simulink model "Van_der_Pol"  (Simulink 9.1)
settings: Solver=VariableStepAuto  StartTime=0.0  StopTime=20  RelTol=1e-3
settings Model: SuppressorTable=22 serialization::archive 11 0 6 0 0 0 0 0  Creator=BEAR  LastModifiedBy=BEAR
settings DataIOCC: SaveFormat=Dataset
settings OptimizationCC: LifeSpan=auto
settings DebuggingCC: UnderspecifiedInitializationDetection=Simplified  MergeDetectMultiDrivingBlocksExec=error  SFUnexpectedBacktrackingDiag=error  SFNoUnconditionalDefaultTransitionDiag=error  SFExecutionAtInitializationDiag=warning
settings HardwareCC: ProdBitPerPointer=64  ProdBitPerSizeT=64  ProdBitPerPtrDiffT=64  ProdLargestAtomicFloat=Float  ProdIntDivRoundTo=Zero  ProdEndianess=LittleEndian  ProdWordSize=64  ProdHWDeviceType=Intel->x86-64 (Windows64)
settings ModelReferenceCC: PropagateSignalLabelsOutOfModel=on
settings CodeAppCC: StateflowObjectComments=off
settings GRTTargetCC: TargetLangStandard=C99 (ISO)  CombineOutputUpdateFcns=on  GRTInterface=off
settings ConfigComp: CovMetricSettings=dwe  CovHtmlReporting=off  CovSaveCumulativeToWorkspaceVar=off  CovSaveSingleToWorkspaceVar=off  CovExternalEMLEnable=on

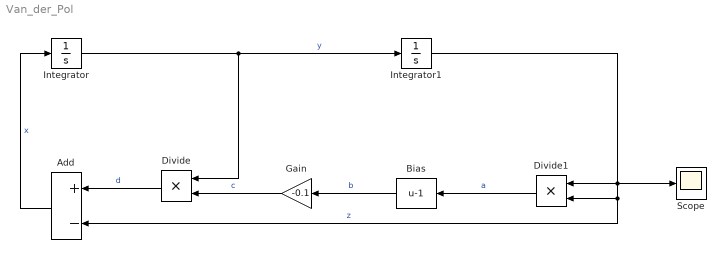
== system Van_der_Pol ==
  Add : Sum  Inputs=+-
  Bias : Bias  Bias=-1
  Divide : Product  Inputs=**
  Divide1 : Product  Inputs=**  SampleTime=6
  Gain : Gain  Gain=-0.1  SampleTime=4
  Integrator : Integrator  InitialCondition=1
  Integrator1 : Integrator  InitialCondition=1
  Scope : Scope
  wires:
  Add/1 -> Integrator/1  "x"
  Divide/1 -> Add/1  "d"
  Integrator/1 -> Divide/1, Integrator1/1  "y"
  Gain/1 -> Divide/2  "c"
  Bias/1 -> Gain/1  "b"
  Divide1/1 -> Bias/1  "a"
  Integrator1/1 -> Scope/1, Divide1/1, Divide1/2, Add/2  "z"
